simulink model "lat747mod9dn"  (Simulink 8.7)
settings: Solver=ode5  SolverMode=SingleTasking  StartTime=0.0  StopTime=50  FixedStep=T  RelTol=1e-6
undefined symbols (not defined in the file): A, B, C, Kd, T
settings Model: Creator=OJ  LastModifiedBy=Soren  ExtModeTrigMode=oneshot  ExtModeArmWhenConnect=off
settings DataIOCC: LimitDataPoints=off  SignalLoggingSaveFormat=ModelDataLogs
settings OptimizationCC: BooleanDataType=off  ExpressionDepthLimit=2147483647  InitFltsAndDblsToZero=on
settings DebuggingCC: SaveWithParameterizedLinksMsg=none  SignalResolutionControl=TryResolveAllWithWarning  MultiTaskCondExecSysMsg=none  FcnCallInpInsideContextMsg=UseLocalSettings  UnconnectedInputMsg=none  UnconnectedOutputMsg=none  UnconnectedLineMsg=none  StateNameClashWarn=warning  StrictBusMsg=Warning
settings HardwareCC: TargetUnknown=on
settings GRTTargetCC: TargetFcnLib=ansi_tfl_tmw.mat  CombineOutputUpdateFcns=off  GRTInterface=on

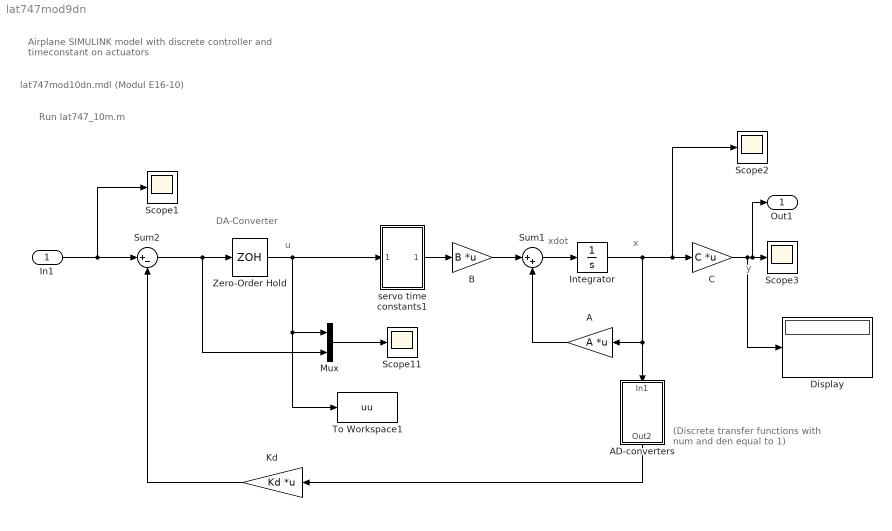
== system lat747mod9dn ==
  note: y
  note: x
  note: xdot
  note: (Discrete transfer functions
      | with num and den equal to 1)
  note: DA-Converter
  note: u
  note: Airplane SIMULINK model with discrete controller
      | and timeconstant on actuators
  note: lat747mod10dn.mdl (Modul E16-10)
  note: Run lat747_10m.m
  In1 : Inport  PortDimensions=2
  A : Gain  Gain=A  Multiplication=Matrix(K*u)  SaturateOnIntegerOverflow=on  OutDataTypeStr=Inherit: Same as input  ParamDataTypeStr=Inherit: Same as input
  AD-converters : Subsystem
  B : Gain  Gain=B  Multiplication=Matrix(K*u)  SaturateOnIntegerOverflow=on  OutDataTypeStr=Inherit: Same as input  ParamDataTypeStr=Inherit: Same as input
  C : Gain  Gain=C  Multiplication=Matrix(K*u)  SaturateOnIntegerOverflow=on  OutDataTypeStr=Inherit: Same as input  ParamDataTypeStr=Inherit: Same as input
  Display : Display
  Integrator : Integrator  InitialCondition=0%[-.050 .02 -.1 .04]'
  Kd : Gain  Gain=Kd  Multiplication=Matrix(K*u)  SampleTime=T  SaturateOnIntegerOverflow=on  OutDataTypeStr=Inherit: Same as input  ParamDataTypeStr=Inherit: Same as input
  Mux : Mux  Inputs=2
  Scope{1..3,11} (4 alike) : Scope
  Sum1 : Sum  Inputs=|++  SaturateOnIntegerOverflow=on  InputSameDT=on  OutDataTypeStr=Inherit: Same as first input
  Sum2 : Sum  Inputs=|+-  SampleTime=T  SaturateOnIntegerOverflow=on  InputSameDT=on  OutDataTypeStr=Inherit: Same as first input
  To Workspace1 : ToWorkspace  VariableName=uu
  Zero-Order Hold : ZeroOrderHold  SampleTime=T
  servo time constants1 : Subsystem
  Out1 : Outport
  wires:
  Integrator/1 -> C/1, Scope2/1, A/1, AD-converters/1(In1)
  Sum1/1 -> Integrator/1
  B/1 -> Sum1/1
  A/1 -> Sum1/2
  C/1 -> Out1/1, Scope3/1, Display/1
  Sum2/1 -> Zero-Order Hold/1, Mux/2
  Zero-Order Hold/1 -> Mux/1, To Workspace1/1, servo time constants1/1(In1)
  Mux/1 -> Scope11/1
  Kd/1 -> Sum2/2
  AD-converters/1(Out2) -> Kd/1
  In1/1 -> Sum2/1, Scope1/1
  servo time constants1/1(Out1) -> B/1

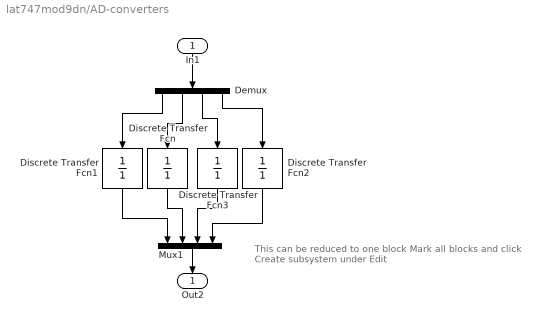
== system lat747mod9dn/AD-converters ==
  note: This can be reduced to one block
      | Mark all blocks and click  Create subsystem under Edit
  In1 : Inport
  Demux : Demux
  Discrete Transfer Fcn{,1..3} (4 alike) : DiscreteTransferFcn  Numerator=1  Denominator=1  SampleTime=T
  Mux1 : Mux
  Out2 : Outport
  wires:
  Demux/2 -> Discrete Transfer Fcn/1
  Demux/4 -> Discrete Transfer Fcn2/1
  Demux/3 -> Discrete Transfer Fcn3/1
  Demux/1 -> Discrete Transfer Fcn1/1
  Discrete Transfer Fcn2/1 -> Mux1/4
  Discrete Transfer Fcn3/1 -> Mux1/3
  Discrete Transfer Fcn/1 -> Mux1/2
  Discrete Transfer Fcn1/1 -> Mux1/1
  In1/1 -> Demux/1
  Mux1/1 -> Out2/1

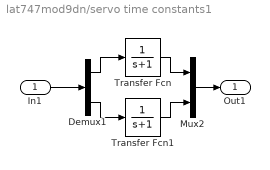
== system lat747mod9dn/servo time constants1 ==
  In1 : Inport
  Demux1 : Demux  Outputs=2
  Mux2 : Mux  Inputs=2
  Transfer Fcn : TransferFcn  Denominator=[1 1]
  Transfer Fcn1 : TransferFcn  Denominator=[1 1]
  Out1 : Outport
  wires:
  Demux1/1 -> Transfer Fcn/1
  Demux1/2 -> Transfer Fcn1/1
  Transfer Fcn/1 -> Mux2/1
  Transfer Fcn1/1 -> Mux2/2
  In1/1 -> Demux1/1
  Mux2/1 -> Out1/1
